simulink model "state_feed"  (R2020b)
settings: Solver=VariableStepAuto  StartTime=0.0  StopTime=10.0  RelTol=1e-3
values from neighbouring files (symbols this model uses):
  alpha = 1    [Reg.m]    (also in State_feed.m = [-(C-D*K)*(A-B*K)^-1*B+D]^-1)
  K = place(A,B,[-1 -7])    [E3_5.m]    (also in E_140421_1.m = place(A,B,[20 -10]); Esempi.m = place(A,B,[-1,-2,-3]); EserciziFinali.m = place(A,B,[20, -10]); Problem_P2.m = 20*log10(m))
libraries: simulink x1
settings Model: Creator=kevin  LastModifiedBy=kevin

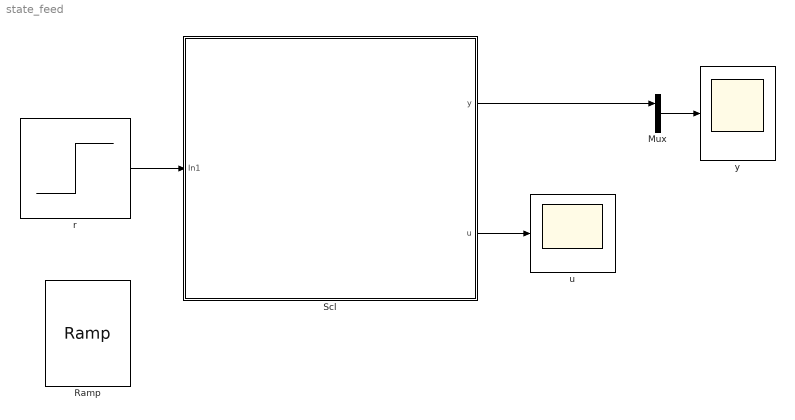
== system state_feed ==
  Mux : Mux  Inputs=2
  Ramp : simulink/Sources/Ramp  slope=1  start=0  InitialOutput=0
  Scl : Subsystem
  r : Step  Time=0  SampleTime=0
  u : Scope
  y : Scope
  wires:
  Scl/1(y) -> Mux/1
  Scl/2(u) -> u/1
  Mux/1 -> y/1
  r/1 -> Scl/1(In1)

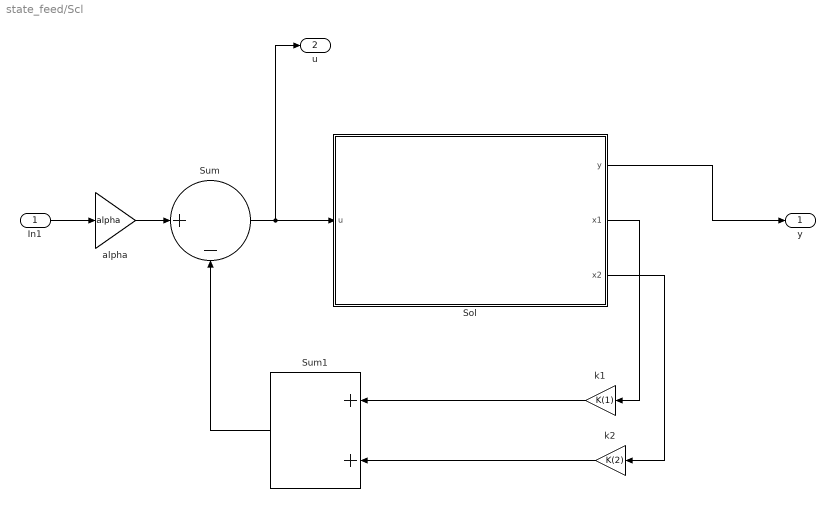
== system state_feed/Scl ==
  In1 : Inport
  Sol : Subsystem
  Sum : Sum  Inputs=|+-
  Sum1 : Sum
  alpha : Gain  Gain=alpha
  k1 : Gain  Gain=K(1)
  k2 : Gain  Gain=K(2)
  y : Outport
  u : Outport  Port=2
  wires:
  Sum/1 -> u/1, Sol/1(u)
  Sol/3(x2) -> k2/1
  Sol/2(x1) -> k1/1
  In1/1 -> alpha/1
  Sol/1(y) -> y/1
  k2/1 -> Sum1/2
  k1/1 -> Sum1/1
  alpha/1 -> Sum/1
  Sum1/1 -> Sum/2

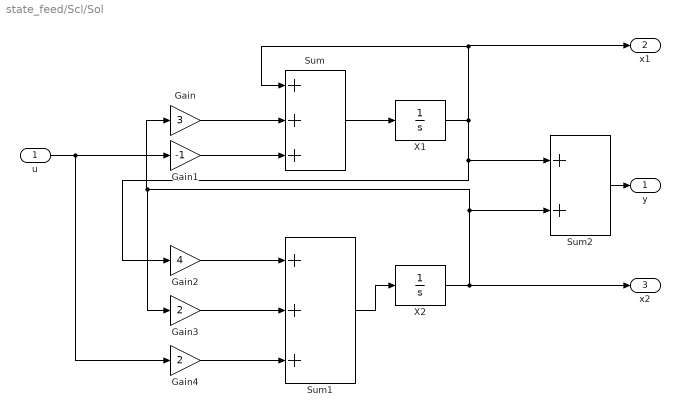
== system state_feed/Scl/Sol ==
  u : Inport
  Gain : Gain  Gain=3
  Gain1 : Gain  Gain=-1
  Gain2 : Gain  Gain=4
  Gain3 : Gain  Gain=2
  Gain4 : Gain  Gain=2
  Sum : Sum  Inputs=+++
  Sum1 : Sum  Inputs=+++
  Sum2 : Sum
  X1 : Integrator
  X2 : Integrator
  y : Outport
  x1 : Outport  Port=2
  x2 : Outport  Port=3
  wires:
  Gain4/1 -> Sum1/3
  Sum/1 -> X1/1
  X2/1 -> x2/1, Sum2/2, Gain3/1, Gain/1
  Gain3/1 -> Sum1/2
  Sum1/1 -> X2/1
  Gain/1 -> Sum/2
  Gain1/1 -> Sum/3
  u/1 -> Gain4/1, Gain1/1
  X1/1 -> Sum2/1, Gain2/1, x1/1, Sum/1
  Gain2/1 -> Sum1/1
  Sum2/1 -> y/1
